simulink model "trajectory_planner"  (R2025b)
settings: configuration reference "MCConfiguration" (kept outside this file)
undefined symbols (not defined in the file): position, trajectory_time
libraries: arsenal x3, simulink x2, dspsigops x1
settings Model: DataDictionary=embeddedBoard_common.sldd  Creator=rpumpo  LastModifiedBy=rpumpo
settings ConfigSetRef: SourceName=MCConfiguration

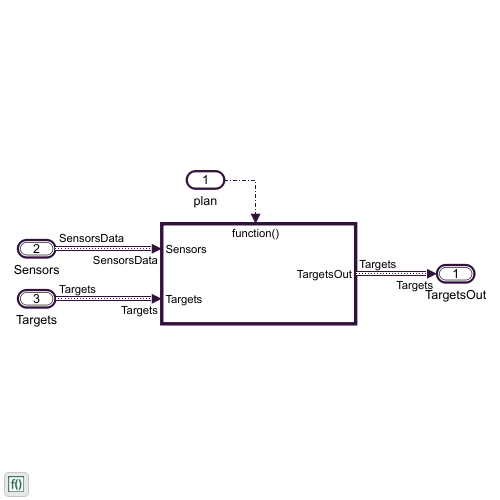
[thumbnail: Simulink's stored preview of the top-level diagram]
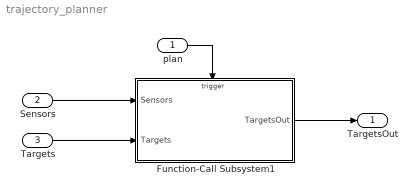
== system trajectory_planner ==
  plan : Inport  SampleTime=0.001  OutputFunctionCall=on
  Sensors : Inport  Port=2  OutDataTypeStr=Bus: SensorsData  BusOutputAsStruct=on
  Targets : Inport  Port=3  OutDataTypeStr=Bus: Targets  BusOutputAsStruct=on
  Function-Call Subsystem1 : Subsystem  TreatAsAtomicUnit=on
  TargetsOut : Outport  OutDataTypeStr=Bus: Targets  BusOutputAsStruct=on
  wires:
  plan/1 -> Function-Call Subsystem1/Trigger
  Sensors/1 -> Function-Call Subsystem1/1(Sensors)
  Targets/1 -> Function-Call Subsystem1/2(Targets)
  Function-Call Subsystem1/1(TargetsOut) -> TargetsOut/1

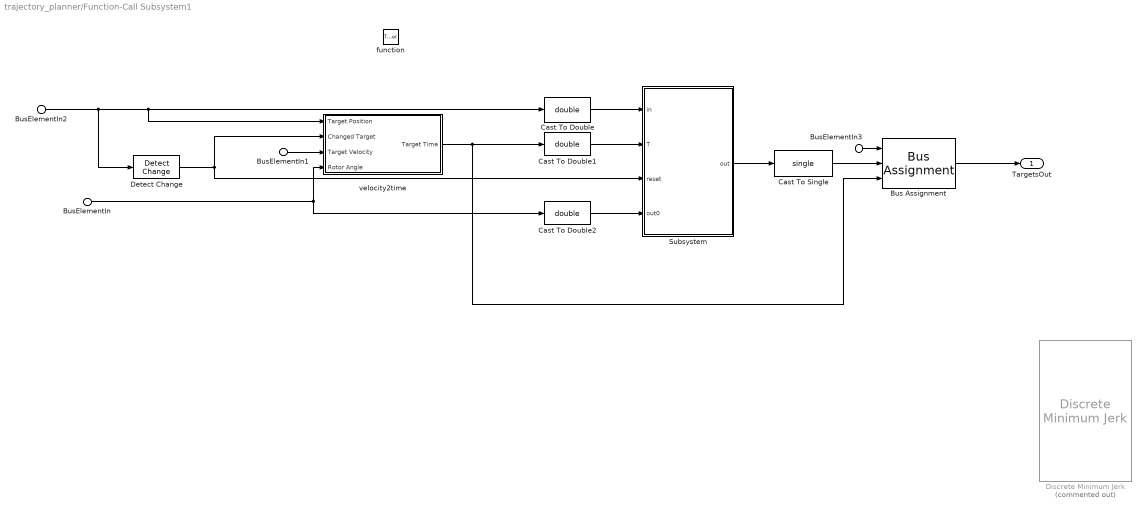
== system trajectory_planner/Function-Call Subsystem1 ==
  BusElementIn : Inport  Description=Mechanical Angle before gearbox  PortName=Sensors  Element=motorsensors.qencoder.rotor_angle
  BusElementIn3 : Inport  Port=2  PortName=Targets
  BusElementIn2 : Inport  Port=2  PortName=Targets  Element=position
  BusElementIn1 : Inport  Port=2  PortName=Targets  Element=velocity
  function : TriggerPort  TriggerType=function-call  VariantControl=(inherit)
  Bus Assignment : BusAssignment  AssignedSignals=position,trajectory_time
  Cast To Double : DataTypeConversion  OutDataTypeStr=double  SaturateOnIntegerOverflow=off  RndMeth=Floor
  Cast To Double1 : DataTypeConversion  OutDataTypeStr=double  SaturateOnIntegerOverflow=off  RndMeth=Floor
  Cast To Double2 : DataTypeConversion  OutDataTypeStr=double  SaturateOnIntegerOverflow=off  RndMeth=Floor
  Cast To Single : DataTypeConversion  OutDataTypeStr=single  SaturateOnIntegerOverflow=off  RndMeth=Floor
  Detect Change : simulink/Logic and Bit Operations/Detect Change  vinit=0  OutDataTypeStr=boolean
  Discrete Minimum Jerk : arsenal/Filters/Discrete Minimum Jerk  Commented=on  Ts=1
      settings: SourceProductName=iCub Tech Arsenal
  Subsystem : Subsystem
  velocity2time : Subsystem
  TargetsOut : Outport  OutDataTypeStr=Bus: Targets
  wires:
  Cast To Double/1 -> Subsystem/1(in)
  Cast To Double1/1 -> Subsystem/2(T)
  Cast To Double2/1 -> Subsystem/4(out0)
  Bus Assignment/1 -> TargetsOut/1
  Subsystem/1(out) -> Cast To Single/1
  BusElementIn1/1 -> velocity2time/3(Target Velocity)
  BusElementIn3/1 -> Bus Assignment/1
  Cast To Single/1 -> Bus Assignment/2
  Detect Change/1 -> velocity2time/2(Changed Target), Subsystem/3(reset)
  velocity2time/1(Target Time) -> Bus Assignment/3, Cast To Double1/1
  BusElementIn2/1 -> Detect Change/1, velocity2time/1(Target Position), Cast To Double/1
  BusElementIn/1 -> Cast To Double2/1, velocity2time/4(Rotor Angle)

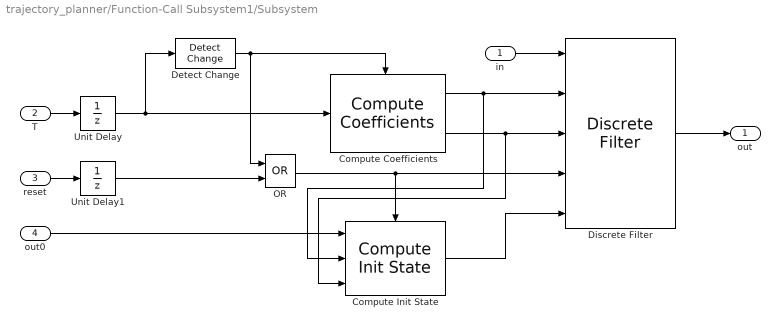
== system trajectory_planner/Function-Call Subsystem1/Subsystem ==
  in : Inport  PortDimensions=1
  T : Inport  Port=2  PortDimensions=1
  reset : Inport  Port=3  PortDimensions=1
  out0 : Inport  Port=4  PortDimensions=1
  Compute Coefficients : arsenal/Filters/Discrete Minimum Jerk/Compute Coefficients  SystemSampleTime=-1  VariantActivationTime=update diagram  EmptyChoice=off  PassThrough=off  PassThroughVariantControl=(default)  EmptyChoiceVariantControl=(default)  AllowFlexibleInterface=on  Latency=0  AutoFrameSizeCalculation=off
      link override Constant: Value=4*Ts_Supervision
      link override Constant6: Value=2*Ts_Supervision^2
      link override Constant7: Value=Ts_Supervision^3
      settings: SourceProductName=iCub Tech Arsenal
  Compute Init State : arsenal/Filters/Discrete Minimum Jerk/Compute Init State  SystemSampleTime=-1  VariantActivationTime=update diagram  EmptyChoice=off  PassThrough=off  PassThroughVariantControl=(default)  EmptyChoiceVariantControl=(default)  AllowFlexibleInterface=on  Latency=0  AutoFrameSizeCalculation=off
  Detect Change : simulink/Logic and Bit Operations/Detect Change  vinit=0  OutDataTypeStr=uint8
  Discrete Filter : DiscreteFilter  NumeratorSource=Input port  DenominatorSource=Input port  InitialStatesSource=Input port  ExternalReset=Rising  a0EqualsOne=on
      settings: InputPortMap=u0,p1,p3,r7,p5
  OR : Logic  Operator=OR  AllPortsSameDT=off  OutDataTypeStr=boolean
  Unit Delay : UnitDelay  SampleTime=-1  HasFrameUpgradeWarning=on
  Unit Delay1 : UnitDelay  SampleTime=-1  HasFrameUpgradeWarning=on
  out : Outport  PortDimensions=1
  wires:
  Detect Change/1 -> OR/1, Compute Coefficients/Trigger
  reset/1 -> Unit Delay1/1
  Compute Init State/1 -> Discrete Filter/5
  Compute Coefficients/1 -> Discrete Filter/2, Compute Init State/2
  out0/1 -> Compute Init State/1
  T/1 -> Unit Delay/1
  OR/1 -> Discrete Filter/4, Compute Init State/Trigger
  Compute Coefficients/2 -> Discrete Filter/3, Compute Init State/3
  Discrete Filter/1 -> out/1
  Unit Delay/1 -> Detect Change/1, Compute Coefficients/1
  in/1 -> Discrete Filter/1
  Unit Delay1/1 -> OR/2

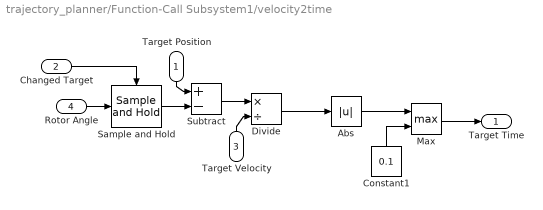
== system trajectory_planner/Function-Call Subsystem1/velocity2time ==
  Target Position : Inport
  Changed Target : Inport  Port=2
  Target Velocity : Inport  Port=3
  Rotor Angle : Inport  Port=4
  Abs : Abs  SaturateOnIntegerOverflow=off
  Constant1 : Constant  Value=0.1  OutDataTypeStr=single
  Divide : Product  Inputs=*/
  Max : MinMax  Function=max  Inputs=2
  Sample and Hold : dspsigops/Sample and Hold  trig=Rising edge  initCond=0  latchinput=off
  Subtract : Sum  Inputs=+-
  Target Time : Outport
  wires:
  Rotor Angle/1 -> Sample and Hold/1
  Target Position/1 -> Subtract/1
  Changed Target/1 -> Sample and Hold/Trigger
  Max/1 -> Target Time/1
  Sample and Hold/1 -> Subtract/2
  Abs/1 -> Max/1
  Constant1/1 -> Max/2
  Subtract/1 -> Divide/1
  Target Velocity/1 -> Divide/2
  Divide/1 -> Abs/1
